simulink model "delay"  (R2015a)
settings: Solver=ode45  StartTime=0.0  StopTime=10.0  RelTol=1e-3
libraries: dspvision x1, dspsnks4 x1
settings Model: Creator=ai  LastModifiedBy=ai

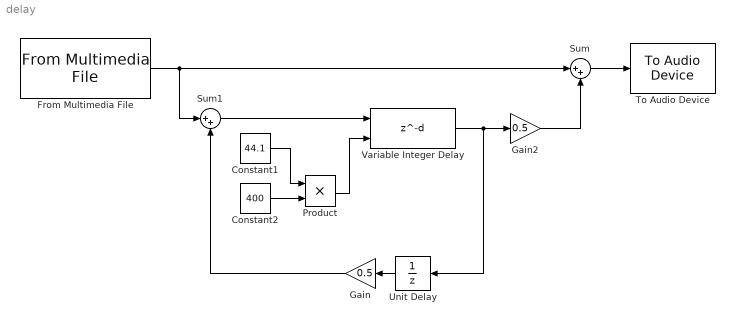
== system delay ==
  Constant1 : Constant  Value=44.1
  Constant2 : Constant  Value=400
  From Multimedia File : dspvision/From Multimedia File  inputFilename=speech_dft.mp3  loop=on  numPlays=inf  outputStreams=Audio only  videoDataType=single  audioDataType=double  inheritSampleTime=on  userDefinedSampleTime=1/30  noAudioOutput=off  isIntensityVideo=off  fourcc=RGB  colorVideoFormat=Separate color signals  outputEOF=off  dataOrg=Column-major  audioFrameSize=1024  computeAudioFrameSize=off  outSamplingMode=Sample based
  Gain : Gain  Gain=0.5
  Gain2 : Gain  Gain=0.5
  Product : Product
  Sum : Sum  Inputs=|++
  Sum1 : Sum  Inputs=|++
  To Audio Device : dspsnks4/To Audio Device  deviceName=Default  inheritSampleRate=on  sampleRate=44100  deviceDatatype=Determine from input data type  autoBufferSize=on  bufferSize=4096  queueDuration=1.0  defaultOutputChannelMapping=on  outputChannelMapping=1:2  outputNumUnderrunSamples=off
  Unit Delay : UnitDelay  SampleTime=-1
  Variable Integer Delay : Delay  DelayLengthSource=Input port  DelayLengthUpperLimit=22050  InputProcessing=Columns as channels (frame based)  UseCircularBuffer=on
      settings: InputPortMap=u0,p1
  wires:
  From Multimedia File/1 -> Sum/1, Sum1/1
  Variable Integer Delay/1 -> Unit Delay/1, Gain2/1
  Sum1/1 -> Variable Integer Delay/1
  Sum/1 -> To Audio Device/1
  Gain/1 -> Sum1/2
  Gain2/1 -> Sum/2
  Constant2/1 -> Product/2
  Product/1 -> Variable Integer Delay/2
  Constant1/1 -> Product/1
  Unit Delay/1 -> Gain/1
